simulink model "smc"  (R2024b)
settings: Solver=ode45  StartTime=0.0  StopTime=100  FixedStep=1e-3  RelTol=1e-4
values from neighbouring files (symbols this model uses):
  alpha = p(10)    [tumor_growth_controlled.m]    (also in tumor_growth_state_controlled.m)
  b1 = p(3)    [tumor_growth_controlled.m]    (also in tumor_growth_state_controlled.m)
  b2 = p(4)    [tumor_growth_controlled.m]    (also in tumor_growth_state_controlled.m)
  c1 = p(5)    [tumor_growth_controlled.m]    (also in tumor_growth_state_controlled.m)
  c2 = p(6)    [tumor_growth_controlled.m]    (also in tumor_growth_state_controlled.m)
  c3 = p(7)    [tumor_growth_controlled.m]    (also in tumor_growth_state_controlled.m)
  c4 = p(8)    [tumor_growth_controlled.m]    (also in tumor_growth_state_controlled.m)
  d1 = p(12)    [tumor_growth_controlled.m]    (also in tumor_growth_state_controlled.m)
  gamma1 = p(13)    [tumor_growth_controlled.m]    (also in tumor_growth_state_controlled.m)
  gamma2 = p(14)    [tumor_growth_controlled.m]    (also in tumor_growth_state_controlled.m)
  gamma3 = p(15)    [tumor_growth_controlled.m]    (also in tumor_growth_state_controlled.m)
  k = p(16)    [tumor_growth_controlled.m]    (also in tumor_growth_state_controlled.m)
  r1 = p(1)    [tumor_growth_controlled.m]    (also in tumor_growth_state_controlled.m)
  r2 = p(2)    [tumor_growth_controlled.m]    (also in tumor_growth_state_controlled.m)
  rho = p(9)    [tumor_growth_controlled.m]    (also in tumor_growth_state_controlled.m)
  s = p(11)    [tumor_growth_controlled.m]    (also in tumor_growth_state_controlled.m)
undefined symbols (not defined in the file or in its folder): epsilon, K, p1, p2, p3, p4, x_0, x_eq
settings Model: Creator=fiore  LastModifiedBy=fiore
settings SolverCC: ZeroCrossAlgorithm=Adaptive
settings DebuggingCC: IgnoredZcDiagnostic=none

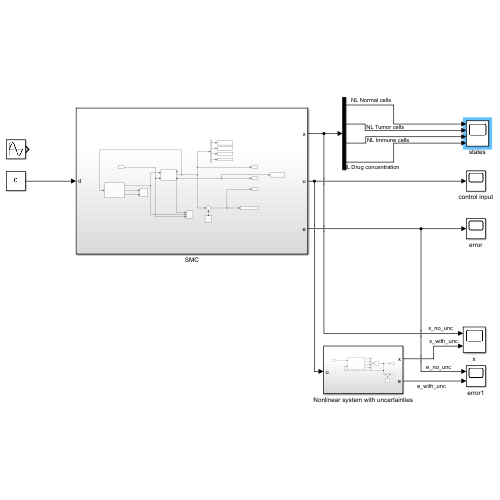
[thumbnail: Simulink's stored preview of the top-level diagram]
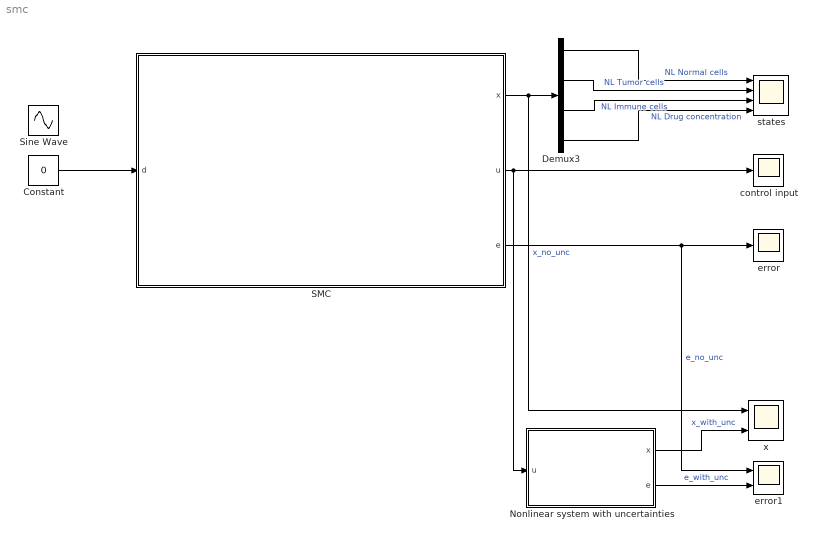
== system smc ==
  Constant : Constant  Value=0
  Demux3 : Demux
  Nonlinear system with uncertainties : Subsystem
  SMC : Subsystem
  Sine Wave : Sin  Amplitude=1.5  Frequency=0.5  SampleTime=0
  control input : Scope
  error : Scope
  error1 : Scope  NumInputPorts=2
  states : Scope  NumInputPorts=4
  x : Scope  NumInputPorts=2
  wires:
  Demux3/1 -> states/1  "NL Normal cells"
  SMC/1(x) -> x/1, Demux3/1  "x_no_unc"
  Demux3/3 -> states/3  "NL Immune cells"
  Demux3/4 -> states/4  "NL Drug concentration"
  Demux3/2 -> states/2  "NL Tumor cells"
  SMC/3(e) -> error/1, error1/1  "e_no_unc"
  SMC/2(u) -> control input/1, Nonlinear system with uncertainties/1(u)
  Nonlinear system with uncertainties/1(x) -> x/2  "x_with_unc"
  Nonlinear system with uncertainties/2(e) -> error1/2  "e_with_unc"
  Constant/1 -> SMC/1(d)

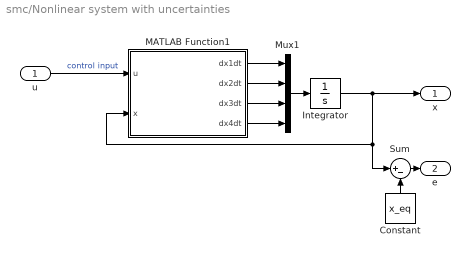
== system smc/Nonlinear system with uncertainties ==
  u : Inport
  Constant : Constant  Value=x_eq
  Integrator : Integrator  InitialCondition=x_0  LimitOutput=on  LowerSaturationLimit=0  ZeroCross=off
  MATLAB Function1 : MATLAB Function  TreatAsAtomicUnit=on
  Mux1 : Mux
  Sum : Sum  Inputs=|+-
  x : Outport
  e : Outport  Port=2
  wires:
  MATLAB Function1/2(dx2dt) -> Mux1/2
  MATLAB Function1/1(dx1dt) -> Mux1/1
  MATLAB Function1/3(dx3dt) -> Mux1/3
  MATLAB Function1/4(dx4dt) -> Mux1/4
  Mux1/1 -> Integrator/1
  Integrator/1 -> x/1, Sum/1, MATLAB Function1/2(x)
  u/1 -> MATLAB Function1/1(u)  "control input"
  Sum/1 -> e/1
  Constant/1 -> Sum/2

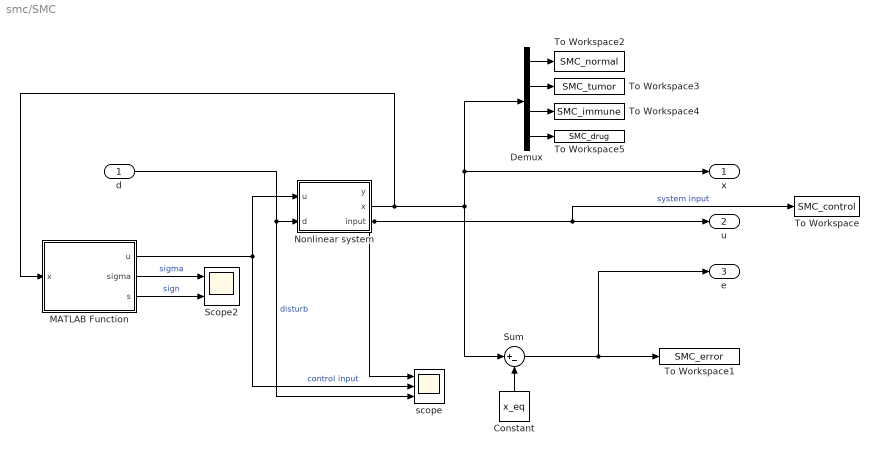
== system smc/SMC ==
  d : Inport
  Constant : Constant  Value=x_eq
  Demux : Demux
  MATLAB Function : MATLAB Function  TreatAsAtomicUnit=on
  Nonlinear system : Subsystem
  Scope2 : Scope  NumInputPorts=2
  Sum : Sum  Inputs=|+-
  To Workspace : ToWorkspace  VariableName=SMC_control  SaveFormat=Timeseries  SampleTime=-1
  To Workspace1 : ToWorkspace  VariableName=SMC_error  SaveFormat=Timeseries  SampleTime=-1
  To Workspace2 : ToWorkspace  VariableName=SMC_normal  SaveFormat=Timeseries  SampleTime=-1
  To Workspace3 : ToWorkspace  VariableName=SMC_tumor  SaveFormat=Timeseries  SampleTime=-1
  To Workspace4 : ToWorkspace  VariableName=SMC_immune  SaveFormat=Timeseries  SampleTime=-1
  To Workspace5 : ToWorkspace  VariableName=SMC_drug  SaveFormat=Timeseries  SampleTime=-1
  scope : Scope  NumInputPorts=3
  x : Outport
  u : Outport  Port=2
  e : Outport  Port=3
  wires:
  MATLAB Function/1(u) -> scope/2, Nonlinear system/1(u)  "control input"
  Sum/1 -> e/1, To Workspace1/1
  MATLAB Function/2(sigma) -> Scope2/1  "sigma"
  Demux/2 -> To Workspace3/1
  Demux/4 -> To Workspace5/1
  Demux/3 -> To Workspace4/1
  MATLAB Function/3(s) -> Scope2/2  "sign"
  Nonlinear system/3(input) -> To Workspace/1, u/1, scope/1  "system input"
  Constant/1 -> Sum/2
  Nonlinear system/2(x) -> x/1, Demux/1, Sum/1, MATLAB Function/1(x)
  Demux/1 -> To Workspace2/1
  d/1 -> scope/3, Nonlinear system/2(d)  "disturb"

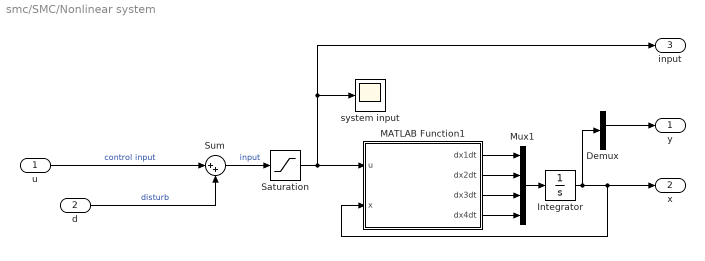
== system smc/SMC/Nonlinear system ==
  u : Inport
  d : Inport  Port=2
  Demux : Demux
  Integrator : Integrator  InitialCondition=x_0  LimitOutput=on  LowerSaturationLimit=0  ZeroCross=off
  MATLAB Function1 : MATLAB Function  TreatAsAtomicUnit=on
  Mux1 : Mux
  Saturation : Saturate  UpperLimit=inf  LowerLimit=0
  Sum : Sum  Inputs=|++
  system input : Scope
  y : Outport
  x : Outport  Port=2
  input : Outport  Port=3
  wires:
  MATLAB Function1/2(dx2dt) -> Mux1/2
  MATLAB Function1/1(dx1dt) -> Mux1/1
  MATLAB Function1/3(dx3dt) -> Mux1/3
  MATLAB Function1/4(dx4dt) -> Mux1/4
  Mux1/1 -> Integrator/1
  Integrator/1 -> x/1, MATLAB Function1/2(x), Demux/1
  Demux/2 -> y/1
  u/1 -> Sum/1  "control input"
  Sum/1 -> Saturation/1  "input"
  Saturation/1 -> system input/1, input/1, MATLAB Function1/1(u)
  d/1 -> Sum/2  "disturb"

== matlab function smc/SMC/MATLAB Function ==
  data: x input; u output; p1 parameter; p2 parameter; k parameter; sigma output; s output; gamma1 parameter; c4 parameter; alpha parameter; gamma3 parameter; gamma2 parameter; d1 parameter; rho parameter; c2 parameter; c3 parameter; c1 parameter; b2 parameter; b1 parameter; r2 parameter; r1 parameter; x_eq parameter; p4 parameter; p3 parameter; K parameter; epsilon parameter
function [u, sigma,s] = SMC(x, p1, p2, k, gamma1, c4, alpha, gamma3, gamma2, d1, rho, c2, c3, c1, b2, b1, r2, r1, x_eq, p4, p3, K, epsilon)  
    x1 = x(1);       % (normal cells)
    x2 = x(2);       % (tumor cells)
    x3 = x(3);       % (immune cells)
    x4 = x(4);       % (drug concentration)

    sigma = p1*(x1 - x_eq(1)) + p2*x2 + p3*(x3 - x_eq(3)) + p4*x4;

    if sigma <-epsilon
        s = -1;
    elseif sigma > epsilon
        s = +1;
    else
        s = sigma/epsilon;
    end 

    f1 = r2 * x1 * (1 - b2 * x1) - c4 * x2 * x1 - gamma1 * x4;
    f2 = r1 * x2 * (1 - b1 * x2) - c2 * x3 * x2 - c3 * x2 * x1 - gamma2 * x4;
    f3 = s + (rho * x3 * x2) / (alpha + x2) - c1 * x3 * x2 - d1 * x3 - gamma3 * x4;   
    f4 = -k*x4;

    lieg = p4;
    lief = p1*f1 + p2*f2 + p3*f3 + p4*f4;

    u = -K*s/lieg - lief/lieg;
end

== matlab function smc/SMC/Nonlinear system/MATLAB Function1 ==
  data: u input; dx1dt output; x input; dx2dt output; r1 parameter; r2 parameter; b1 parameter; b2 parameter; c1 parameter; c3 parameter; c2 parameter; c4 parameter; rho parameter; alpha parameter; s parameter; d1 parameter; dx3dt output; gamma1 parameter; gamma2 parameter; gamma3 parameter; dx4dt output; k parameter
function [dx1dt,dx2dt,dx3dt, dx4dt] = tumor_growth(u,x,r1, r2, b1, b2, c1, c3, c2, c4, rho, alpha, s, d1, gamma1, gamma2, gamma3, k)

    x1 = x(1);       % (normal cells)
    x2 = x(2);       % (tumor cells)
    x3 = x(3);       % (immune cells)
    x4 = x(4);       % (drug concentration)
    
    dx1dt = r2 * x1 * (1 - b2 * x1) - c4 * x2 * x1 - gamma1 * x4;
    dx2dt = r1 * x2 * (1 - b1 * x2) - c2 * x3 * x2 - c3 * x2 * x1 - gamma2 * x4;
    dx3dt = s + (rho * x3 * x2) / (alpha + x2) - c1 * x3 * x2 - d1 * x3 - gamma3 * x4;   
    dx4dt = u - k*x4;
end

== matlab function smc/Nonlinear system with uncertainties/MATLAB Function1 ==
  data: u input; dx1dt output; x input; dx2dt output; r1 parameter; r2 parameter; b1 parameter; b2 parameter; c1 parameter; c3 parameter; c2 parameter; c4 parameter; rho parameter; alpha parameter; s parameter; d1 parameter; dx3dt output; gamma1 parameter; gamma2 parameter; gamma3 parameter; dx4dt output; k parameter
function [dx1dt,dx2dt,dx3dt, dx4dt] = tumor_growth(u,x,r1, r2, b1, b2, c1, c3, c2, c4, rho, alpha, s, d1, gamma1, gamma2, gamma3, k)

    c1_real = c1*(1+0.5);
    c4_real = c4*(1+0.5);

    x1 = x(1);       % (normal cells)
    x2 = x(2);       % (tumor cells)
    x3 = x(3);       % (immune cells)
    x4 = x(4);       % (drug concentration)
    
    dx1dt = r2 * x1 * (1 - b2 * x1) - c4_real * x2 * x1 - gamma1 * x4;
    dx2dt = r1 * x2 * (1 - b1 * x2) - c2 * x3 * x2 - c3 * x2 * x1 - gamma2 * x4;
    dx3dt = s + (rho * x3 * x2) / (alpha + x2) - c1_real * x3 * x2 - d1 * x3 - gamma3 * x4;   
    dx4dt = u - k*x4;
end
